simulink model "conv5x5_video_ex"  (Simulink 7.7)
settings: Solver=VariableStepDiscrete  SolverMode=SingleTasking  StartTime=0.0  StopTime=1000  RelTol=1e-3
undefined symbols (not defined in the file or in its folder): xrbsImage_r3
libraries: xbsIndex_r4 x204, xrbsImage_r4 x1, xbsCopyrightNotice_r4 x1
(part 1 of 3)
settings Model: Creator=alexc  LastModifiedBy=douangp
settings DataIOCC: SignalLoggingName=sigsOut
settings OptimizationCC: InlineParams=on  InitFltsAndDblsToZero=on
settings DebuggingCC: SaveWithParameterizedLinksMsg=none  SignalResolutionControl=TryResolveAllWithWarning  SolverPrmCheckMsg=none  MultiTaskDSMMsg=warning  MultiTaskCondExecSysMsg=none  StrictBusMsg=None
settings HardwareCC: TargetUnknown=on
settings RTWCC: IncludeERTFirstTime=on
settings GRTTargetCC: TargetFcnLib=ansi_tfl_tmw.mat

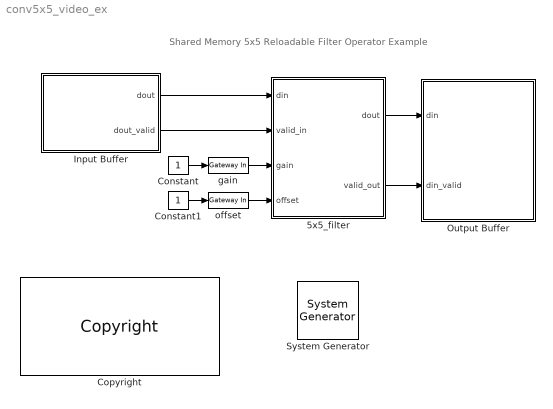
== system conv5x5_video_ex ==
  note: Shared Memory 5x5 Reloadable Filter Operator Example
  " System Generator" : xbsIndex_r4/ System Generator  Tag=genX  SystemSampleTime=-1  xilinxfamily=kintex7  part=xc7k325t  speed=-2  package=ffg900  synthesis_tool=XST  clock_wrapper=Clock Enables  directory=./netlist  proj_type=Project Navigator  Synth_file=XST Defaults  Impl_file=ISE Defaults  testbench=off  simulink_period=1/5  sysclk_period=20  dcm_input_clock_period=100  incr_netlist=off  trim_vbits=Everywhere in SubSystem  dbl_ovrd=According to Block Masks  core_generation=According to Block Masks  run_coregen=off  deprecated_control=off  eval_field=0  block_type=sysgen
      settings: block_version=9.2.00
  5x5_filter : Subsystem
  Constant : Constant
  Constant1 : Constant
  Copyright : xbsCopyrightNotice_r4/Copyright  copyrighttext="Copyright (c) 2011  by  Xilinx, Inc. All rights reserved.<br><br>This file contains proprietary, confidential information of Xilinx, Inc., is distributed under license from Xilinx, Inc., and may be used, copied and/or disclosed only pursuant to the terms of a valid license agreement with Xilinx, Inc. Xilinx hereby grants you a license to use this file solely for design, simulation, implementation and creation of design files limited to Xilinx devices or technologies. Use with non-Xilinx devices or technologies is expressly prohibited and immediately terminates your license unless covered by a separate agreement.<br><br>Xilinx is providing this design, code, or information \"as-is\" solely for use in developing programs and solutions for Xilinx devices, with no obligation on the part of Xilinx to provide support. By providing this design, code, or information as one possible implementation of this feature, application or standard, Xilinx is making no representation that this implementation is free from any claims of infringement. You are responsible for obtaining any rights you may require for your implementation. Xilinx expressly disclaims any warranty whatsoever with respect to the adequacy of the implementation, including but not limited to any warranties or representations that this implementation is free from claims of infringement, implied warranties of merchantability or fitness for a particular purpose.<br><br>Xilinx products are not intended for use in life support appliances, devices, or systems. Use in such applications is expressly prohibited.<br><br>Any modifications that are made to the Source Code are done at the user's sole risk and will be unsupported.<br><br>This copyright and support notice must be retained as part of this text at all times. (c) Copyright 1995-2011 Xilinx, Inc. All rights reserved."  block_type=copyright
      settings: block_version=10.1.00
      settings: infoedit=|
      | Copyright(C) 2008 by  Xilinx, Inc. All rights reserved.<br>
      | <br>
      | This file contains proprietary, confidential information of Xilinx, Inc., is distributed under license
      | from Xilinx, Inc., and may be used, copied and/or disclosed only pursuant to the terms of a valid license
      | agreement with Xilinx, Inc. Xilinx hereby grants you a license to use this file solely for design,
      | simulation, implementation and creation of design files limited to Xilinx devices or technologies. Use
      | with non-Xilinx devices or technologies is expressly prohibited and immediately terminates your license
      | unless covered by a separate agreement.<br>
      | <br>
      | Xilinx is providing this design, code, or information "as-is" solely for use in developing programs and
      | solutions for Xilinx devices, with no obligation on the part of Xilinx to provide support. By providing
      | this design, code, or information as one possible implementation of this feature, application or standard,
      | Xilinx is making no representation that this implementation is free from any claims of infringement. You
      | are responsible for obtaining any rights you may require for your implementation. Xilinx expressly disclaims
      | any warranty whatsoever with respect to the adequacy of the implementation, including but not limited to any
      | warranties or representations that this implementation is free from claims of infringement, implied warranties
      | of merchantability or fitness for a particular purpose.<br>
      | <br>
      | Xilinx products are not intended for use in life support appliances, devices, or systems. Use in such
      | applications is expressly prohibited.<br>
      | <br>
      | Any modifications that are made to the Source Code are done at the user's sole risk and will be unsupported.<br>
      | <br>
      | This copyright and support notice must be retained as part of this text at all times.
      | (c) Copyright 1995-2008 Xilinx, Inc. All rights reserved.
  Input Buffer : Subsystem  mask{smName='Foo', smDepth=128*128, smWidth=8}
      mask prompts: smName "Shared Memory Name"; smDepth "Shared Memory Depth"; smWidth "Shared Memory Width"
  Output Buffer : Subsystem  mask{smName='Bar', smDepth=128*128}
      mask prompts: smName "Shared Memory Name"; smDepth "Shared Memory Depth"
  gain : xbsIndex_r4/Gateway In  gui_display_data_type=Fixed-point  arith_type="Signed  (2's comp)"  n_bits=20  bin_pt=17  preci_type=Single  exp_width=8  frac_width=24  quantization="Round  (unbiased: +/- Inf)"  overflow=Saturate  period=1  dbl_ovrd=off  timing_constraint=None  locs_specified=off  LOCs={}  hdl_port=on  block_type=gatewayin
      settings: infoedit="Gateway in block.  Converts inputs of type Simulink integer, double and fixed point to  Xilinx fixed point type.<P><P>Hardware notes:  In hardware these blocks become top level input ports."  xl_area=[0, 0, 0, 0, 0, 0, 0]  block_version=VER_STRING_GOES_HERE
  offset : xbsIndex_r4/Gateway In  gui_display_data_type=Fixed-point  arith_type=Unsigned  n_bits=10  bin_pt=0  preci_type=Single  exp_width=8  frac_width=24  quantization="Round  (unbiased: +/- Inf)"  overflow=Saturate  period=1  dbl_ovrd=off  timing_constraint=None  locs_specified=off  LOCs={}  hdl_port=on  block_type=gatewayin
      settings: infoedit="Gateway in block.  Converts inputs of type Simulink integer, double and fixed point to  Xilinx fixed point type.<P><P>Hardware notes:  In hardware these blocks become top level input ports."  xl_area=[0, 0, 0, 0, 0, 0, 0]  block_version=VER_STRING_GOES_HERE
  wires:
  Input Buffer/1(dout) -> 5x5_filter/1(din)
  Constant/1 -> gain/1
  Constant1/1 -> offset/1
  5x5_filter/1(dout) -> Output Buffer/1(din)
  5x5_filter/2(valid_out) -> Output Buffer/2(din_valid)
  Input Buffer/2(dout_valid) -> 5x5_filter/2(valid_in)
  gain/1 -> 5x5_filter/3(gain)
  offset/1 -> 5x5_filter/4(offset)

== system conv5x5_video_ex/5x5_filter ==
  din : Inport
  valid_in : Inport  Port=2
  gain : Inport  Port=3
  offset : Inport  Port=4
  5x5Filter : Subsystem  AncestorBlock=xrbsImage_r3/5x5Filter  mask(5x5 Filter){maskNum=Smooth, coef_n_bits=6, coef_bin_pt=0, smpl_n_bits=8, smpl_bin_pt=0, smpl_period=1, maskVal=0, maskDiv=0}
      mask prompts: maskNum "5x5 Mask"; coef_n_bits "Number of Bits per Coefficient"; coef_bin_pt "Binary Point for Coefficient"; smpl_n_bits "Number of Bits per Input Sample"; smpl_bin_pt "Binary Point for Input Samples"; smpl_period "Sample Period"; maskVal "Mask Value"; maskDiv "Mask Division"
      mask help: The Xilinx 5x5 Filter reference block is implemented using 5 n-tap MAC FIR Filters. Nine different 2-D filters have been provided to filter grayscale images.
      mask init:
      | [bg,fg] = xlcmap('XBlock',0);
      | iPos = get_param(gcb,'Position');
      | iWidth=iPos(3)-iPos(1); iHeight=iPos(4)-iPos(2);
      | iCx=iWidth/2;
      | iCy=iHeight/2;
      | [logoX, logoY] = xlogo(iPos);
      | 
      | % Different 5x5 Filters 
      | %  by default edge is used
      | 
      | edge = [ 0  0  0  0 0; ...
      |          0 -1 -1 -1 0; ...
      |          0 -1  8 -1 0; ...
      |          0 -1 -1 -1 0; ...
      |          0  0  0  0 0];
      | edgeDiv = 1;
      | 
      | sobelX = [ 0  0  0  0 0; ...
      |            0 -1  0  1 0; ...
      |            0 -2  0  2 0; ...
      |            0 -1  0  1 0; ...
      |            0  0  0  0 0];
      | sobelXDiv = 1;
      | 
      | sobelY = [ 0  0  0  0 0; ...
      |            0  1  2  1 0; ...
      |            0  0  0  0 0; ...
      |            0 -1  2 -1 0; ...
      |            0  0  0  0 0];
      | sobelYDiv = 1;
      | 
      | sobelXY = [ 0  0  0  0 0; ...
      |             0  0 -1 -1 0; ...
      |             0  1  0 -1 0; ...
      |             0  1  1  0 0; ...
      |             0  0  0  0 0];
      | sobelXYDiv = 1;
      | 
      | blur = [ 1  1  1  1 1; ...
      |          1  0  0  0 1; ...
      |          1  0  0  0 1; ...
      |          1  0  0  0 1; ...
      |          1  1  1  1 1];
      | blurDiv = 1/16;
      | 
      | smooth = [ 1  1  1  1 1; ...
      |            1  5  5  5 1; ...
      |            1  5 44  5 1; ...
      |            1  5  5  5 1; ...
      |            1  1  1  1 1];
      | smoothDiv = 1/100;
      | 
      | sharpen = [ 0  0  0  0 0; ...
      |             0 -2 -2 -2 0; ...
      |             0 -2 32 -2 0; ...
      |             0 -2 -2 -2 0; ...
      |             0  0  0  0 0];
      | sharpenDiv = 1/16;
      | 
      | 
      | gaussian = [1 1 2 1 1; ...
      |             1 2 4 2 1; ...
      |             2 4 8 4 2; ...
      |             1 2 4 2 1; ...
      |             1 1 2 1 1];
      | gaussianDiv = 1/52;
      | 
      | identity = [ 0  0  0  0 0; ...
      |              0  0  0  0 0; ...
      |              0  0  1  0 0; ...
      |              0  0  0  0 0; ...
      |              0  0  0  0 0];
      | identityDiv = 1;
      | 
      | maskVal = zeros(5,5,5);
      | maskVal(:,:,1) = edge;
      | maskVal(:,:,2) = sobelX;
      | maskVal(:,:,3) = sobelY;
      | maskVal(:,:,4) = sobelXY;
      | maskVal(:,:,5) = blur;
      | maskVal(:,:,6) = smooth;
      | maskVal(:,:,7) = sharpen;
      | maskVal(:,:,8) = gaussian;
      | maskVal(:,:,9) = identity;
      | 
      | maskDiv = [edgeDiv sobelXDiv sobelYDiv sobelXYDiv blurDiv smoothDiv sharpenDiv gaussianDiv identityDiv];
      mask Help: web(xlhtmldoclink('5x5Filter'));
      mask StyleString: popup(Edge|Sobel X|Sobel Y|Sobel X-Y|Blur|Smooth|Sharpen|Gaussian|Identity),edit,edit,edit,edit,edit,edit,edit
      mask Display:
      | patch([0 iWidth iWidth 0],[0 0 iHeight iHeight] , bg);
      | patch(logoX,logoY , fg);
      | port_label('input',1,'Line1');
      | port_label('input',2,'Line2');
      | port_label('input',3,'Line3');
      | port_label('input',4,'Line4');
      | port_label('input',5,'Line5');
      | port_label('input',6,'Load');
      | port_label('input',7,'Coef');
      | port_label('input',8,'Gain');
      | port_label('output',1,'out');
      | plot([0 0 iWidth iWidth 0], [0 iHeight iHeight 0 0]);
  Register16 : xbsIndex_r4/Register  init=0  rst=off  en=off  dbl_ovrd=off  block_type=register
      settings: xl_area=[4 8 0 0 0 0 0]  block_version=VER_STRING_GOES_HERE
  Register2 : xbsIndex_r4/Register  init=0  rst=off  en=off  dbl_ovrd=off  block_type=register
      settings: xl_area=[4 8 0 0 0 0 0]  block_version=VER_STRING_GOES_HERE
  Virtex2 5 Line Buffer1 : xrbsImage_r4/Virtex2 5 Line Buffer  SystemSampleTime=-1  line_size=128  cst=1
      link override Virtex2 Line Buffer/Single Port RAM: block_version=8.2
      link override Virtex2 Line Buffer1/Single Port RAM: block_version=8.2
      link override Virtex2 Line Buffer2/Single Port RAM: block_version=8.2
      link override Virtex2 Line Buffer3/Single Port RAM: block_version=8.2
  coefficient_memory : Subsystem  mask{width=6, bin_pt=0, period=1/5}
      mask prompts: width "Coefficient Width"; bin_pt "Coefficient Binary Point"; period "Sample Period"
  valid_generator : Subsystem
  dout : Outport
  valid_out : Outport  Port=2
  wires:
  valid_in/1 -> valid_generator/1(valid_in)
  Register16/1 -> Virtex2 5 Line Buffer1/1
  5x5Filter/1(Out1) -> Register2/1
  Virtex2 5 Line Buffer1/1 -> 5x5Filter/1(Line1)
  Virtex2 5 Line Buffer1/2 -> 5x5Filter/2(Line2)
  Virtex2 5 Line Buffer1/3 -> 5x5Filter/3(Line3)
  Virtex2 5 Line Buffer1/4 -> 5x5Filter/4(Line4)
  Virtex2 5 Line Buffer1/5 -> 5x5Filter/5(Line5)
  Register2/1 -> dout/1
  din/1 -> Register16/1
  offset/1 -> valid_generator/2(offset)
  valid_generator/1(valid_out) -> valid_out/1
  gain/1 -> 5x5Filter/8(gain)
  coefficient_memory/1(load) -> 5x5Filter/6(load)
  coefficient_memory/2(coef) -> 5x5Filter/7(coef)

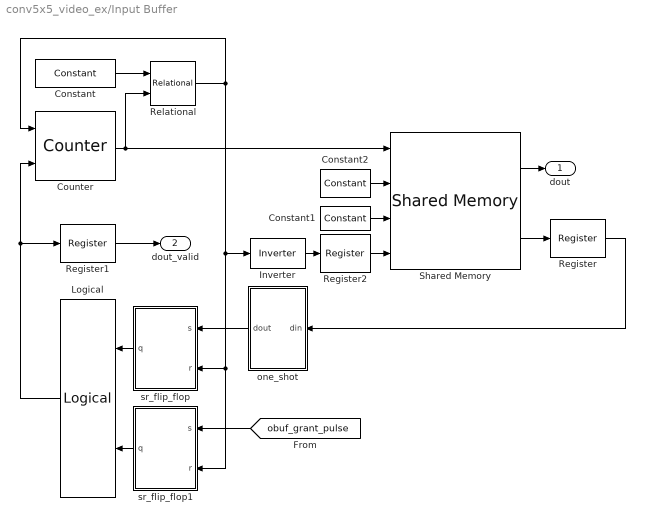
== system conv5x5_video_ex/Input Buffer ==
  Constant : xbsIndex_r4/Constant  const=smDepth-1  gui_display_data_type=Fixed-point  arith_type=Unsigned  n_bits=ceil(log2(smDepth))  bin_pt=0  preci_type=Single  exp_width=8  frac_width=24  explicit_period=on  period=1  equ=P=C  opselect=C  inp2=PCIN>>17  opr=+  inp1=P  carry=CIN  dbl_ovrd=off  block_type=constant
      settings: block_version=VER_STRING_GOES_HERE
  Constant1 : xbsIndex_r4/Constant  const=0  gui_display_data_type=Fixed-point  arith_type=Boolean  n_bits=1  bin_pt=0  preci_type=Single  exp_width=8  frac_width=24  explicit_period=off  period=1  equ=P=C  opselect=C  inp2=PCIN>>17  opr=+  inp1=P  carry=CIN  dbl_ovrd=off  block_type=constant
      settings: block_version=VER_STRING_GOES_HERE
  Constant2 : xbsIndex_r4/Constant  const=0  gui_display_data_type=Fixed-point  arith_type=Unsigned  n_bits=smWidth  bin_pt=0  preci_type=Single  exp_width=8  frac_width=24  explicit_period=off  period=1  equ=P=C  opselect=C  inp2=PCIN>>17  opr=+  inp1=P  carry=CIN  dbl_ovrd=off  block_type=constant
      settings: block_version=VER_STRING_GOES_HERE
  Counter : xbsIndex_r4/Counter  cnt_type=Free Running  cnt_to=Inf  operation=Up  start_count=0  cnt_by_val=1  arith_type=Unsigned  n_bits=ceil(log2(smDepth))  bin_pt=0  load_pin=off  rst=on  en=on  explicit_period=on  period=1  dbl_ovrd=off  use_behavioral_HDL=off  implementation=Fabric  use_rpm=off  block_type=counter
      settings: infoedit="Configurable up, down and up/down counter.<P><P>Hardware notes: Free running counters are the least expensive in hardware.  A count limited counter is implemented by combining a counter with a comparator."  xl_area=[0, 0, 0, 0, 0, 0, 0]  block_version=VER_STRING_GOES_HERE
  Inverter : xbsIndex_r4/Inverter  en=off  latency=0  dbl_ovrd=off  block_type=inv
      settings: xl_area=[0, 0, 0, 0, 0, 0, 0]  block_version=VER_STRING_GOES_HERE
  Logical : xbsIndex_r4/Logical  logical_function=AND  inputs=2  en=off  latency=0  precision=Full  arith_type=Unsigned  n_bits=8  bin_pt=2  align_bp=on  dbl_ovrd=off  block_type=logical
      settings: xl_area=[0, 0, 0, 0, 0, 0, 0]  block_version=VER_STRING_GOES_HERE
  Register : xbsIndex_r4/Register  init=0  rst=off  en=off  dbl_ovrd=off  block_type=register
      settings: xl_area=[0, 0, 0, 0, 0, 0, 0]  block_version=VER_STRING_GOES_HERE
  Register1 : xbsIndex_r4/Register  init=0  rst=off  en=off  dbl_ovrd=off  block_type=register
      settings: xl_area=[0, 0, 0, 0, 0, 0, 0]  block_version=VER_STRING_GOES_HERE
  Register2 : xbsIndex_r4/Register  init=0  rst=off  en=off  dbl_ovrd=off  block_type=register
      settings: xl_area=[0, 0, 0, 0, 0, 0, 0]  block_version=VER_STRING_GOES_HERE
  Relational : xbsIndex_r4/Relational  mode=a=b  en=off  latency=0  dbl_ovrd=off  block_type=relational
      settings: xl_area=[0, 0, 0, 0, 0, 0, 0]  block_version=VER_STRING_GOES_HERE
  Shared Memory : xbsIndex_r4/Shared Memory  shared_memory_name=smName  depth=smDepth  ownership=Locally Owned and Initialized  initVector=0:255  en=off  mutex=Lockable  mode=Read and Write  write_mode=Read After Write  time_out=0  latency=1  explicit_data_type=off  gui_display_data_type=Fixed-point  arith_type=Unsigned  n_bits=0  bin_pt=0  preci_type=Single  implementation=Block RAM  use_rpm=off  block_type=shmem
      settings: AttributesFormatString=<< %<shared_memory_name> >>  xl_area=[0, 0, 0, 0, 0, 0, 0]  block_version=VER_STRING_GOES_HERE
  one_shot : Subsystem
  sr_flip_flop : Subsystem
  sr_flip_flop1 : Subsystem
  dout : Outport
  dout_valid : Outport  Port=2
  wires:
  Shared Memory/2 -> Register/1
  Counter/1 -> Shared Memory/1, Relational/2
  Constant/1 -> Relational/1
  Relational/1 -> Inverter/1, sr_flip_flop/2(r), sr_flip_flop1/2(r), Counter/1
  Inverter/1 -> Register2/1
  Register2/1 -> Shared Memory/4
  Constant1/1 -> Shared Memory/3
  Constant2/1 -> Shared Memory/2
  [obuf_grant_pulse] -> sr_flip_flop1/1(s)
  one_shot/1(dout) -> sr_flip_flop/1(s)
  sr_flip_flop1/1(q) -> Logical/2
  sr_flip_flop/1(q) -> Logical/1
  Logical/1 -> Counter/2, Register1/1
  Register/1 -> one_shot/1(din)
  Register1/1 -> dout_valid/1
  Shared Memory/1 -> dout/1

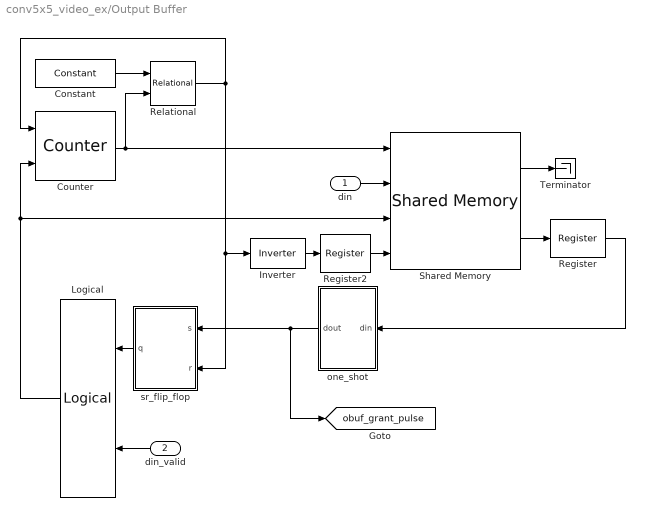
== system conv5x5_video_ex/Output Buffer ==
  din : Inport
  din_valid : Inport  Port=2
  Constant : xbsIndex_r4/Constant  const=smDepth-1  gui_display_data_type=Fixed-point  arith_type=Unsigned  n_bits=ceil(log2(smDepth))  bin_pt=0  preci_type=Single  exp_width=8  frac_width=24  explicit_period=on  period=1  equ=P=C  opselect=C  inp2=PCIN>>17  opr=+  inp1=P  carry=CIN  dbl_ovrd=off  block_type=constant
      settings: block_version=VER_STRING_GOES_HERE
  Counter : xbsIndex_r4/Counter  cnt_type=Free Running  cnt_to=Inf  operation=Up  start_count=0  cnt_by_val=1  arith_type=Unsigned  n_bits=ceil(log2(smDepth))  bin_pt=0  load_pin=off  rst=on  en=on  explicit_period=on  period=1  dbl_ovrd=off  use_behavioral_HDL=off  implementation=Fabric  use_rpm=off  block_type=counter
      settings: infoedit="Configurable up, down and up/down counter.<P><P>Hardware notes: Free running counters are the least expensive in hardware.  A count limited counter is implemented by combining a counter with a comparator."  xl_area=[0, 0, 0, 0, 0, 0, 0]  block_version=VER_STRING_GOES_HERE
  Inverter : xbsIndex_r4/Inverter  en=off  latency=0  dbl_ovrd=off  block_type=inv
      settings: xl_area=[0, 0, 0, 0, 0, 0, 0]  block_version=VER_STRING_GOES_HERE
  Logical : xbsIndex_r4/Logical  logical_function=AND  inputs=2  en=off  latency=0  precision=Full  arith_type=Unsigned  n_bits=8  bin_pt=2  align_bp=on  dbl_ovrd=off  block_type=logical
      settings: xl_area=[0, 0, 0, 0, 0, 0, 0]  block_version=VER_STRING_GOES_HERE
  Register : xbsIndex_r4/Register  init=0  rst=off  en=off  dbl_ovrd=off  block_type=register
      settings: xl_area=[0, 0, 0, 0, 0, 0, 0]  block_version=VER_STRING_GOES_HERE
  Register2 : xbsIndex_r4/Register  init=0  rst=off  en=off  dbl_ovrd=off  block_type=register
      settings: xl_area=[0, 0, 0, 0, 0, 0, 0]  block_version=VER_STRING_GOES_HERE
  Relational : xbsIndex_r4/Relational  mode=a=b  en=off  latency=0  dbl_ovrd=off  block_type=relational
      settings: xl_area=[0, 0, 0, 0, 0, 0, 0]  block_version=VER_STRING_GOES_HERE
  Shared Memory : xbsIndex_r4/Shared Memory  shared_memory_name=smName  depth=smDepth  ownership=Locally Owned and Initialized  initVector=0  en=off  mutex=Lockable  mode=Read and Write  write_mode=Read After Write  time_out=0  latency=1  explicit_data_type=off  gui_display_data_type=Fixed-point  arith_type=Unsigned  n_bits=0  bin_pt=0  preci_type=Single  implementation=Block RAM  use_rpm=off  block_type=shmem
      settings: AttributesFormatString=<< %<shared_memory_name> >>  xl_area=[0, 0, 0, 0, 0, 0, 0]  block_version=VER_STRING_GOES_HERE
  Terminator : Terminator
  one_shot : Subsystem
  sr_flip_flop : Subsystem
  tag scope: obuf_grant_pulse=global
  wires:
  Shared Memory/1 -> Terminator/1
  Register/1 -> one_shot/1(din)
  Logical/1 -> Counter/2, Shared Memory/3
  sr_flip_flop/1(q) -> Logical/1
  one_shot/1(dout) -> sr_flip_flop/1(s), [obuf_grant_pulse]
  Register2/1 -> Shared Memory/4
  Inverter/1 -> Register2/1
  Relational/1 -> Counter/1, Inverter/1, sr_flip_flop/2(r)
  Constant/1 -> Relational/1
  Counter/1 -> Relational/2, Shared Memory/1
  Shared Memory/2 -> Register/1
  din_valid/1 -> Logical/2
  din/1 -> Shared Memory/2

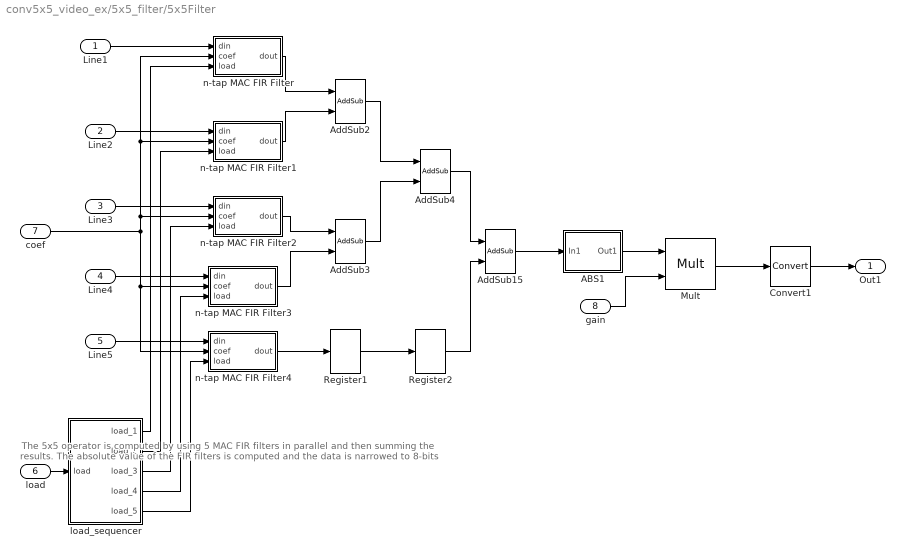
== system conv5x5_video_ex/5x5_filter/5x5Filter ==
  note: The 5x5 operator is computed by using 5 MAC FIR filters in parallel and then
      | summing the results.  The absolute value of the FIR filters is computed
      | and the data is narrowed to 8-bits
  Line1 : Inport
  Line2 : Inport  Port=2
  Line3 : Inport  Port=3
  Line4 : Inport  Port=4
  Line5 : Inport  Port=5
  load : Inport  Port=6
  coef : Inport  Port=7
  gain : Inport  Port=8
  ABS1 : Subsystem
  AddSub{2..4,15} (4 alike) : xbsIndex_r4/AddSub  mode=Addition  use_carryin=off  use_carryout=off  en=off  latency=1  precision=Full  arith_type=Unsigned  n_bits=8  bin_pt=2  quantization=Truncate  overflow=Wrap  dbl_ovrd=off  use_behavioral_HDL=off  hw_selection=Fabric  pipelined=off  use_rpm=off  block_type=addsub
      settings: xl_area=[0, 0, 0, 0, 0, 0, 0]  block_version=VER_STRING_GOES_HERE
  Convert1 : xbsIndex_r4/Convert  gui_display_data_type=Fixed-point  arith_type=Unsigned  n_bits=8  bin_pt=0  float_type=Single  exp_bits=8  fraction_bits=24  quantization=Truncate  overflow=Saturate  en=off  latency=1  dbl_ovrd=off  pipeline=off  block_type=convert
      settings: infoedit=The input is presented at the output after quantization and overflow effects.<P><P>Hardware notes: Additional hardware is used when rounding or saturation is selected and output width is less than the input width.  xl_area=[0, 0, 0, 0, 0, 0, 0]  block_version=VER_STRING_GOES_HERE
  Mult : xbsIndex_r4/Mult  precision=Full  arith_type="Signed  (2's comp)"  n_bits=8  bin_pt=2  quantization=Truncate  overflow=Wrap  en=off  latency=5  dbl_ovrd=off  use_behavioral_HDL=off  opt=Speed  use_embedded=on  optimum_pipeline=off  pipeline=on  use_rpm=off  placement_style=Rectangular shape  block_type=mult
      settings: infoedit=Multiplies two values.<P><P>Hardware notes: To use the internal pipeline stage of the dedicated multiplier you must select 'Pipeline to Greatest Extent Possible'.  xl_area=[0, 0, 0, 0, 0, 0, 0]  block_version=VER_STRING_GOES_HERE
  Register1 : xbsIndex_r4/Register  init=0  rst=off  en=off  dbl_ovrd=off  block_type=register
      settings: xl_area=[0, 0, 0, 0, 0, 0, 0]  block_version=VER_STRING_GOES_HERE
  Register2 : xbsIndex_r4/Register  init=0  rst=off  en=off  dbl_ovrd=off  block_type=register
      settings: xl_area=[0, 0, 0, 0, 0, 0, 0]  block_version=VER_STRING_GOES_HERE
  load_sequencer : Subsystem  mask{num_coef=5}
      mask prompts: num_coef "Number of Coefficients"
  n-tap MAC FIR Filter : Subsystem  AncestorBlock=xrbsDSP_r3/n-tap MAC FIR Filter  mask(n-tap MAC FIR Filter){coef=maskVal(1,5:-1:1,maskNum), coef_n_bits=coef_n_bits, coef_bin_pt=coef_bin_pt, smpl_n_bits=smpl_n_bits, smpl_bin_pt=smpl_bin_pt, smpl_period=smpl_period}
      mask prompts: coef "Coefficients"; coef_n_bits "Number of Bits per Coefficient"; coef_bin_pt "Binary Point for Coefficient"; smpl_n_bits "Number of Bits per Input Sample"; smpl_bin_pt "Binary Point for Input Samples"; smpl_period "Input Sample Period"
      mask help: MAC-based FIR filter with n coefficients.
      mask init:
      | dstr = sprintf('%d tap',length(coef));
      | 
      | [bg,fg] = xlcmap('XBlock',0);
      | iPos = get_param(gcb,'Position');
      | iWidth=iPos(3)-iPos(1); iHeight=iPos(4)-iPos(2);
      | iCx=iWidth/2;
      | iCy=iHeight/2;
      | [logoX, logoY] = xlogo(iPos);
      mask Help: web(xlhtmldoclink('n-tap MAC FIR Filter'));
      mask Display:
      | patch([0 iWidth iWidth 0],[0 0 iHeight iHeight] , bg);
      | patch(logoX,logoY, fg);
      | text(iCx/1.8,iCy+2,dstr);
      | text(iCx/2.0-4,iCy-10,'MAC FIR');
      | plot([0 0 iWidth iWidth 0], [0 iHeight iHeight 0 0]);
  n-tap MAC FIR Filter1 : Subsystem  AncestorBlock=xrbsDSP_r3/n-tap MAC FIR Filter  mask(n-tap MAC FIR Filter){coef=maskVal(2,5:-1:1,maskNum), coef_n_bits=coef_n_bits, coef_bin_pt=coef_bin_pt, smpl_n_bits=smpl_n_bits, smpl_bin_pt=smpl_bin_pt, smpl_period=smpl_period}
      mask prompts: coef "Coefficients"; coef_n_bits "Number of Bits per Coefficient"; coef_bin_pt "Binary Point for Coefficient"; smpl_n_bits "Number of Bits per Input Sample"; smpl_bin_pt "Binary Point for Input Samples"; smpl_period "Input Sample Period"
      mask help: MAC-based FIR filter with n coefficients.
      mask init: same as conv5x5_video_ex/5x5_filter/5x5Filter/n-tap MAC FIR Filter
      mask Help: web(xlhtmldoclink('n-tap MAC FIR Filter'));
      mask Display:
      | patch([0 iWidth iWidth 0],[0 0 iHeight iHeight] , bg);
      | patch(logoX,logoY, fg);
      | text(iCx/1.8,iCy+2,dstr);
      | text(iCx/2.0-4,iCy-10,'MAC FIR');
      | plot([0 0 iWidth iWidth 0], [0 iHeight iHeight 0 0]);
  n-tap MAC FIR Filter2 : Subsystem  AncestorBlock=xrbsDSP_r3/n-tap MAC FIR Filter  mask(n-tap MAC FIR Filter){coef=maskVal(3,5:-1:1,maskNum), coef_n_bits=coef_n_bits, coef_bin_pt=coef_bin_pt, smpl_n_bits=smpl_n_bits, smpl_bin_pt=smpl_bin_pt, smpl_period=smpl_period}
      mask prompts: coef "Coefficients"; coef_n_bits "Number of Bits per Coefficient"; coef_bin_pt "Binary Point for Coefficient"; smpl_n_bits "Number of Bits per Input Sample"; smpl_bin_pt "Binary Point for Input Samples"; smpl_period "Input Sample Period"
      mask help: MAC-based FIR filter with n coefficients.
      mask init: same as conv5x5_video_ex/5x5_filter/5x5Filter/n-tap MAC FIR Filter
      mask Help: web(xlhtmldoclink('n-tap MAC FIR Filter'));
      mask Display:
      | patch([0 iWidth iWidth 0],[0 0 iHeight iHeight] , bg);
      | patch(logoX,logoY, fg);
      | text(iCx/1.8,iCy+2,dstr);
      | text(iCx/2.0-4,iCy-10,'MAC FIR');
      | plot([0 0 iWidth iWidth 0], [0 iHeight iHeight 0 0]);
  n-tap MAC FIR Filter3 : Subsystem  AncestorBlock=xrbsDSP_r3/n-tap MAC FIR Filter  mask(n-tap MAC FIR Filter){coef=maskVal(4,5:-1:1,maskNum), coef_n_bits=coef_n_bits, coef_bin_pt=coef_bin_pt, smpl_n_bits=smpl_n_bits, smpl_bin_pt=smpl_bin_pt, smpl_period=smpl_period}
      mask prompts: coef "Coefficients"; coef_n_bits "Number of Bits per Coefficient"; coef_bin_pt "Binary Point for Coefficient"; smpl_n_bits "Number of Bits per Input Sample"; smpl_bin_pt "Binary Point for Input Samples"; smpl_period "Input Sample Period"
      mask help: MAC-based FIR filter with n coefficients.
      mask init: same as conv5x5_video_ex/5x5_filter/5x5Filter/n-tap MAC FIR Filter
      mask Help: web(xlhtmldoclink('n-tap MAC FIR Filter'));
      mask Display:
      | patch([0 iWidth iWidth 0],[0 0 iHeight iHeight] , bg);
      | patch(logoX,logoY, fg);
      | text(iCx/1.8,iCy+2,dstr);
      | text(iCx/2.0-4,iCy-10,'MAC FIR');
      | plot([0 0 iWidth iWidth 0], [0 iHeight iHeight 0 0]);
  n-tap MAC FIR Filter4 : Subsystem  AncestorBlock=xrbsDSP_r3/n-tap MAC FIR Filter  mask(n-tap MAC FIR Filter){coef=maskVal(5,5:-1:1,maskNum), coef_n_bits=coef_n_bits, coef_bin_pt=coef_bin_pt, smpl_n_bits=smpl_n_bits, smpl_bin_pt=smpl_bin_pt, smpl_period=smpl_period}
      mask prompts: coef "Coefficients"; coef_n_bits "Number of Bits per Coefficient"; coef_bin_pt "Binary Point for Coefficient"; smpl_n_bits "Number of Bits per Input Sample"; smpl_bin_pt "Binary Point for Input Samples"; smpl_period "Input Sample Period"
      mask help: MAC-based FIR filter with n coefficients.
      mask init: same as conv5x5_video_ex/5x5_filter/5x5Filter/n-tap MAC FIR Filter
      mask Help: web(xlhtmldoclink('n-tap MAC FIR Filter'));
      mask Display:
      | patch([0 iWidth iWidth 0],[0 0 iHeight iHeight] , bg);
      | patch(logoX,logoY, fg);
      | text(iCx/1.8,iCy+2,dstr);
      | text(iCx/2.0-4,iCy-10,'MAC FIR');
      | plot([0 0 iWidth iWidth 0], [0 iHeight iHeight 0 0]);
  Out1 : Outport
  wires:
  Line1/1 -> n-tap MAC FIR Filter/1(din)
  Line2/1 -> n-tap MAC FIR Filter1/1(din)
  Line4/1 -> n-tap MAC FIR Filter3/1(din)
  Line5/1 -> n-tap MAC FIR Filter4/1(din)
  n-tap MAC FIR Filter/1(dout) -> AddSub2/1
  n-tap MAC FIR Filter1/1(dout) -> AddSub2/2
  n-tap MAC FIR Filter2/1(dout) -> AddSub3/1
  n-tap MAC FIR Filter3/1(dout) -> AddSub3/2
  AddSub2/1 -> AddSub4/1
  AddSub3/1 -> AddSub4/2
  n-tap MAC FIR Filter4/1(dout) -> Register1/1
  Register1/1 -> Register2/1
  AddSub15/1 -> ABS1/1(In1)
  AddSub4/1 -> AddSub15/1
  Register2/1 -> AddSub15/2
  Mult/1 -> Convert1/1
  ABS1/1(Out1) -> Mult/1
  Convert1/1 -> Out1/1
  gain/1 -> Mult/2
  load/1 -> load_sequencer/1(load)
  Line3/1 -> n-tap MAC FIR Filter2/1(din)
  load_sequencer/1(load_1) -> n-tap MAC FIR Filter/3(load)
  load_sequencer/2(load_2) -> n-tap MAC FIR Filter1/3(load)
  load_sequencer/3(load_3) -> n-tap MAC FIR Filter2/3(load)
  load_sequencer/4(load_4) -> n-tap MAC FIR Filter3/3(load)
  load_sequencer/5(load_5) -> n-tap MAC FIR Filter4/3(load)
  coef/1 -> n-tap MAC FIR Filter/2(coef), n-tap MAC FIR Filter1/2(coef), n-tap MAC FIR Filter2/2(coef), n-tap MAC FIR Filter3/2(coef), n-tap MAC FIR Filter4/2(coef)

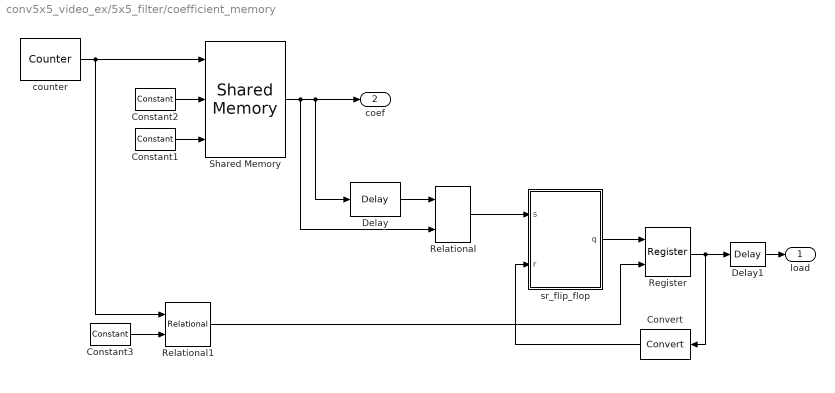
== system conv5x5_video_ex/5x5_filter/coefficient_memory ==
  Constant1 : xbsIndex_r4/Constant  const=0  gui_display_data_type=Fixed-point  arith_type=Boolean  n_bits=width  bin_pt=bin_pt  preci_type=Single  exp_width=8  frac_width=24  explicit_period=off  period=1  equ=P=C  opselect=C  inp2=PCIN>>17  opr=+  inp1=P  carry=CIN  dbl_ovrd=off  block_type=constant
      settings: block_version=VER_STRING_GOES_HERE
  Constant2 : xbsIndex_r4/Constant  const=0  gui_display_data_type=Fixed-point  arith_type=Signed (2's comp)  n_bits=width  bin_pt=bin_pt  preci_type=Single  exp_width=8  frac_width=24  explicit_period=off  period=1  equ=P=C  opselect=C  inp2=PCIN>>17  opr=+  inp1=P  carry=CIN  dbl_ovrd=off  block_type=constant
      settings: block_version=VER_STRING_GOES_HERE
  Constant3 : xbsIndex_r4/Constant  const=24  gui_display_data_type=Fixed-point  arith_type=Unsigned  n_bits=5  bin_pt=0  preci_type=Single  exp_width=8  frac_width=24  explicit_period=off  period=1  equ=P=C  opselect=C  inp2=PCIN>>17  opr=+  inp1=P  carry=CIN  dbl_ovrd=off  block_type=constant
      settings: block_version=VER_STRING_GOES_HERE
  Convert : xbsIndex_r4/Convert  gui_display_data_type=Fixed-point  arith_type=Boolean  n_bits=8  bin_pt=6  float_type=Single  exp_bits=8  fraction_bits=24  quantization=Truncate  overflow=Wrap  en=off  latency=0  dbl_ovrd=off  pipeline=off  block_type=convert
      settings: infoedit=The input is presented at the output after quantization and overflow effects.<P><P>Hardware notes: Additional hardware is used when rounding or saturation is selected and output width is less than the input width.  xl_area=[0, 0, 0, 0, 0, 0, 0]  block_version=VER_STRING_GOES_HERE
  Delay : xbsIndex_r4/Delay  rst=off  infoeditControl=Selection of Reset will increase slice count due to use of real FFs and instead of SRLs  en=off  latency=25  dbl_ovrd=off  reg_retiming=off  block_type=delay
      settings: infoedit="Delay line having  configurable length.<P><P>Hardware notes: A delay line is a chain, each link of which is an SRL16 followed by a flip-flop. If register retiming is enabled, the delay line is a chain of flip-flops."  xl_area=[0, 0, 0, 0, 0, 0, 0]  block_version=VER_STRING_GOES_HERE
  Delay1 : xbsIndex_r4/Delay  rst=off  infoeditControl=Selection of Reset will increase slice count due to use of real FFs and instead of SRLs  en=off  latency=1  dbl_ovrd=off  reg_retiming=off  block_type=delay
      settings: infoedit="Delay line having  configurable length.<P><P>Hardware notes: A delay line is a chain, each link of which is an SRL16 followed by a flip-flop. If register retiming is enabled, the delay line is a chain of flip-flops."  xl_area=[0, 0, 0, 0, 0, 0, 0]  block_version=VER_STRING_GOES_HERE
  Register : xbsIndex_r4/Register  init=0  rst=off  en=on  dbl_ovrd=off  block_type=register
      settings: xl_area=[0, 0, 0, 0, 0, 0, 0]  block_version=VER_STRING_GOES_HERE
  Relational : xbsIndex_r4/Relational  mode=a!=b  en=off  latency=0  dbl_ovrd=off  block_type=relational
      settings: xl_area=[0, 0, 0, 0, 0, 0, 0]  block_version=VER_STRING_GOES_HERE
  Relational1 : xbsIndex_r4/Relational  mode=a=b  en=off  latency=0  dbl_ovrd=off  block_type=relational
      settings: xl_area=[0, 0, 0, 0, 0, 0, 0]  block_version=VER_STRING_GOES_HERE
  Shared Memory : xbsIndex_r4/Shared Memory  shared_memory_name='coef_buffer'  depth=32  ownership=Locally Owned and Initialized  initVector=0  en=off  mutex=Unprotected  mode=Read and Write  write_mode=Read After Write  time_out=0  latency=1  explicit_data_type=off  gui_display_data_type=Fixed-point  arith_type=Unsigned  n_bits=0  bin_pt=0  preci_type=Single  implementation=Block RAM  use_rpm=off  block_type=shmem
      settings: AttributesFormatString=Shared as %<shared_memory_name>  xl_area=[0, 0, 0, 0, 0, 0, 0]  block_version=VER_STRING_GOES_HERE
  counter : xbsIndex_r4/Counter  cnt_type=Count Limited  cnt_to=24  operation=Up  start_count=0  cnt_by_val=1  arith_type=Unsigned  n_bits=5  bin_pt=0  load_pin=off  rst=off  en=off  explicit_period=on  period=period  dbl_ovrd=off  use_behavioral_HDL=off  implementation=Fabric  use_rpm=off  block_type=counter
      settings: infoedit="Configurable up, down and up/down counter.<P><P>Hardware notes: Free running counters are the least expensive in hardware.  A count limited counter is implemented by combining a counter with a comparator."  xl_area=[0, 0, 0, 0, 0, 0, 0]  block_version=VER_STRING_GOES_HERE
  sr_flip_flop : Subsystem
  load : Outport
  coef : Outport  Port=2
  wires:
  Register/1 -> Delay1/1, Convert/1
  Delay1/1 -> load/1
  sr_flip_flop/1(q) -> Register/1
  Relational1/1 -> Register/2
  Constant3/1 -> Relational1/2
  Relational/1 -> sr_flip_flop/1(s)
  Delay/1 -> Relational/1
  Shared Memory/1 -> Relational/2, coef/1, Delay/1
  Constant1/1 -> Shared Memory/3
  counter/1 -> Relational1/1, Shared Memory/1
  Constant2/1 -> Shared Memory/2
  Convert/1 -> sr_flip_flop/2(r)

== system conv5x5_video_ex/5x5_filter/valid_generator ==
  valid_in : Inport
  offset : Inport  Port=2
  ASR : xbsIndex_r4/Addressable Shift Register  infer_latency=on  depth=2  initVector=[0]  en=off  dbl_ovrd=off  use_behavioral_HDL=off  Optimization=Resource  use_rpm=on  block_type=addrsr
      settings: infoedit="Delay of configurable length.  Any element in the delay line can be addressed and driven onto the output port.<P><P>Hardware notes: Implemented using SRL16s.  If a Virtex-II device is used, multiple SRLC16s are cascaded together."  xl_area=[0, 0, 0, 0, 0, 0, 0]  block_version=VER_STRING_GOES_HERE
  Register : xbsIndex_r4/Register  init=0  rst=off  en=off  dbl_ovrd=off  block_type=register
      settings: xl_area=[0, 0, 0, 0, 0, 0, 0]  block_version=VER_STRING_GOES_HERE
  Register1 : xbsIndex_r4/Register  init=0  rst=off  en=on  dbl_ovrd=off  block_type=register
      settings: xl_area=[0, 0, 0, 0, 0, 0, 0]  block_version=VER_STRING_GOES_HERE
  one_shot : Subsystem
  valid_out : Outport
  wires:
  valid_in/1 -> Register/1, one_shot/1(din)
  Register/1 -> ASR/1
  ASR/1 -> valid_out/1
  Register1/1 -> ASR/2
  offset/1 -> Register1/1
  one_shot/1(dout) -> Register1/2

== system conv5x5_video_ex/Input Buffer/one_shot ==
  din : Inport
  Inverter : xbsIndex_r4/Inverter  en=off  latency=0  dbl_ovrd=off  block_type=inv
      settings: xl_area=[0, 0, 0, 0, 0, 0, 0]  block_version=VER_STRING_GOES_HERE
  Logical : xbsIndex_r4/Logical  logical_function=AND  inputs=2  en=off  latency=0  precision=Full  arith_type=Unsigned  n_bits=8  bin_pt=2  align_bp=on  dbl_ovrd=off  block_type=logical
      settings: xl_area=[0, 0, 0, 0, 0, 0, 0]  block_version=VER_STRING_GOES_HERE
  Register1 : xbsIndex_r4/Register  init=0  rst=off  en=off  dbl_ovrd=off  block_type=register
      settings: xl_area=[0, 0, 0, 0, 0, 0, 0]  block_version=VER_STRING_GOES_HERE
  dout : Outport
  wires:
  din/1 -> Register1/1, Logical/1
  Register1/1 -> Inverter/1
  Inverter/1 -> Logical/2
  Logical/1 -> dout/1

== system conv5x5_video_ex/Input Buffer/sr_flip_flop ==
  s : Inport
  r : Inport  Port=2
  Constant2 : xbsIndex_r4/Constant  const=1  gui_display_data_type=Fixed-point  arith_type=Boolean  n_bits=1  bin_pt=0  preci_type=Single  exp_width=8  frac_width=24  explicit_period=off  period=1  equ=P=C  opselect=C  inp2=PCIN>>17  opr=+  inp1=P  carry=CIN  dbl_ovrd=off  block_type=constant
      settings: block_version=VER_STRING_GOES_HERE
  Register1 : xbsIndex_r4/Register  init=0  rst=on  en=on  dbl_ovrd=off  block_type=register
      settings: xl_area=[0, 0, 0, 0, 0, 0, 0]  block_version=VER_STRING_GOES_HERE
  q : Outport
  wires:
  Register1/1 -> q/1
  Constant2/1 -> Register1/1
  r/1 -> Register1/2
  s/1 -> Register1/3

== system conv5x5_video_ex/Input Buffer/sr_flip_flop1 ==
  s : Inport
  r : Inport  Port=2
  Constant2 : xbsIndex_r4/Constant  const=1  gui_display_data_type=Fixed-point  arith_type=Boolean  n_bits=1  bin_pt=0  preci_type=Single  exp_width=8  frac_width=24  explicit_period=off  period=1  equ=P=C  opselect=C  inp2=PCIN>>17  opr=+  inp1=P  carry=CIN  dbl_ovrd=off  block_type=constant
      settings: block_version=VER_STRING_GOES_HERE
  Register1 : xbsIndex_r4/Register  init=0  rst=on  en=on  dbl_ovrd=off  block_type=register
      settings: xl_area=[0, 0, 0, 0, 0, 0, 0]  block_version=VER_STRING_GOES_HERE
  q : Outport
  wires:
  s/1 -> Register1/3
  r/1 -> Register1/2
  Constant2/1 -> Register1/1
  Register1/1 -> q/1

== system conv5x5_video_ex/Output Buffer/one_shot ==
  din : Inport
  Inverter : xbsIndex_r4/Inverter  en=off  latency=0  dbl_ovrd=off  block_type=inv
      settings: xl_area=[0, 0, 0, 0, 0, 0, 0]  block_version=VER_STRING_GOES_HERE
  Logical : xbsIndex_r4/Logical  logical_function=AND  inputs=2  en=off  latency=0  precision=Full  arith_type=Unsigned  n_bits=8  bin_pt=2  align_bp=on  dbl_ovrd=off  block_type=logical
      settings: xl_area=[0, 0, 0, 0, 0, 0, 0]  block_version=VER_STRING_GOES_HERE
  Register1 : xbsIndex_r4/Register  init=0  rst=off  en=off  dbl_ovrd=off  block_type=register
      settings: xl_area=[0, 0, 0, 0, 0, 0, 0]  block_version=VER_STRING_GOES_HERE
  dout : Outport
  wires:
  Logical/1 -> dout/1
  Inverter/1 -> Logical/2
  Register1/1 -> Inverter/1
  din/1 -> Logical/1, Register1/1

== system conv5x5_video_ex/Output Buffer/sr_flip_flop ==
  s : Inport
  r : Inport  Port=2
  Constant2 : xbsIndex_r4/Constant  const=1  gui_display_data_type=Fixed-point  arith_type=Boolean  n_bits=1  bin_pt=0  preci_type=Single  exp_width=8  frac_width=24  explicit_period=off  period=1  equ=P=C  opselect=C  inp2=PCIN>>17  opr=+  inp1=P  carry=CIN  dbl_ovrd=off  block_type=constant
      settings: block_version=VER_STRING_GOES_HERE
  Register1 : xbsIndex_r4/Register  init=0  rst=on  en=on  dbl_ovrd=off  block_type=register
      settings: xl_area=[0, 0, 0, 0, 0, 0, 0]  block_version=VER_STRING_GOES_HERE
  q : Outport
  wires:
  s/1 -> Register1/3
  r/1 -> Register1/2
  Constant2/1 -> Register1/1
  Register1/1 -> q/1

== system conv5x5_video_ex/5x5_filter/5x5Filter/ABS1 ==
  In1 : Inport
  Mux : xbsIndex_r4/Mux  inputs=2  en=off  latency=1  precision=Full  arith_type=Unsigned  n_bits=8  bin_pt=0  quantization=Truncate  overflow=Saturate  dbl_ovrd=off  block_type=mux
      settings: xl_area=[0, 0, 0, 0, 0, 0, 0]  block_version=VER_STRING_GOES_HERE
  Negate : xbsIndex_r4/Negate  precision=Full  arith_type=Unsigned  n_bits=8  bin_pt=2  quantization=Truncate  overflow=Wrap  en=off  latency=1  dbl_ovrd=off  block_type=negate
      settings: xl_area=[0, 0, 0, 0, 0, 0, 0]  block_version=VER_STRING_GOES_HERE
  Register1 : xbsIndex_r4/Register  init=0  rst=off  en=off  dbl_ovrd=off  block_type=register
      settings: xl_area=[0, 0, 0, 0, 0, 0, 0]  block_version=VER_STRING_GOES_HERE
  Register2 : xbsIndex_r4/Register  init=0  rst=off  en=off  dbl_ovrd=off  block_type=register
      settings: xl_area=[0, 0, 0, 0, 0, 0, 0]  block_version=VER_STRING_GOES_HERE
  Slice : xbsIndex_r4/Slice  nbits=1  boolean_output=off  mode=Upper Bit Location + Width  bit1=0  base1=MSB of Input  bit0=0  base0=LSB of Input  dbl_ovrd=off  block_type=slice
      settings: infoedit="Extracts a given range of bits from each input sample and presents it at the output.  The output type is ordinarily unsigned with binary point at zero, but can be Boolean when the slice is one bit wide.<P><P>Hardware notes: In hardware this block costs nothing."  block_version=VER_STRING_GOES_HERE
  Out1 : Outport
  wires:
  Register1/1 -> Mux/2
  Register2/1 -> Mux/1
  Mux/1 -> Out1/1
  In1/1 -> Register1/1, Slice/1, Negate/1
  Negate/1 -> Mux/3
  Slice/1 -> Register2/1

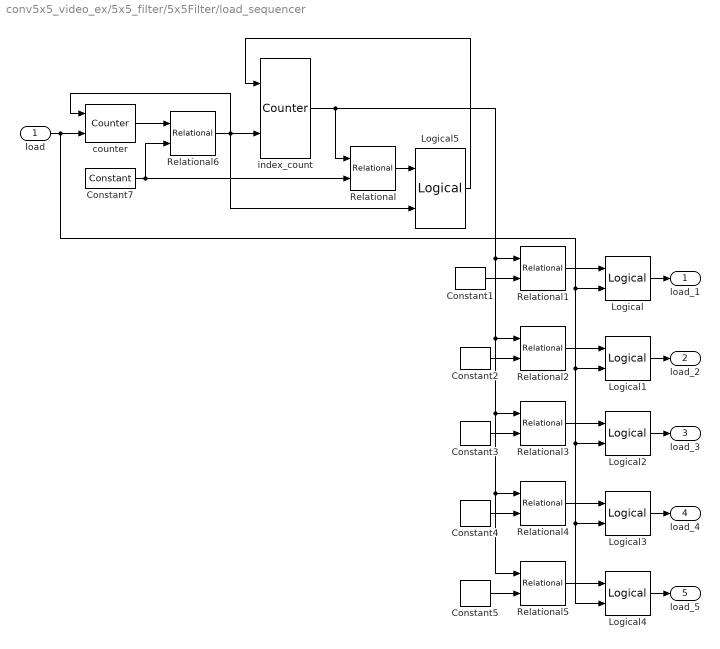
== system conv5x5_video_ex/5x5_filter/5x5Filter/load_sequencer ==
  load : Inport
  Constant1 : xbsIndex_r4/Constant  const=0  gui_display_data_type=Fixed-point  arith_type=Unsigned  n_bits=ceil(log2(num_coef))  bin_pt=0  preci_type=Single  exp_width=8  frac_width=24  explicit_period=off  period=1  equ=P=C  opselect=C  inp2=PCIN>>17  opr=+  inp1=P  carry=CIN  dbl_ovrd=off  block_type=constant
      settings: block_version=VER_STRING_GOES_HERE
  Constant2 : xbsIndex_r4/Constant  const=1  gui_display_data_type=Fixed-point  arith_type=Unsigned  n_bits=ceil(log2(num_coef))  bin_pt=0  preci_type=Single  exp_width=8  frac_width=24  explicit_period=off  period=1  equ=P=C  opselect=C  inp2=PCIN>>17  opr=+  inp1=P  carry=CIN  dbl_ovrd=off  block_type=constant
      settings: block_version=VER_STRING_GOES_HERE
  Constant3 : xbsIndex_r4/Constant  const=2  gui_display_data_type=Fixed-point  arith_type=Unsigned  n_bits=ceil(log2(num_coef))  bin_pt=0  preci_type=Single  exp_width=8  frac_width=24  explicit_period=off  period=1  equ=P=C  opselect=C  inp2=PCIN>>17  opr=+  inp1=P  carry=CIN  dbl_ovrd=off  block_type=constant
      settings: block_version=VER_STRING_GOES_HERE
  Constant4 : xbsIndex_r4/Constant  const=3  gui_display_data_type=Fixed-point  arith_type=Unsigned  n_bits=ceil(log2(num_coef))  bin_pt=0  preci_type=Single  exp_width=8  frac_width=24  explicit_period=off  period=1  equ=P=C  opselect=C  inp2=PCIN>>17  opr=+  inp1=P  carry=CIN  dbl_ovrd=off  block_type=constant
      settings: block_version=VER_STRING_GOES_HERE
  Constant5 : xbsIndex_r4/Constant  const=4  gui_display_data_type=Fixed-point  arith_type=Unsigned  n_bits=ceil(log2(num_coef))  bin_pt=0  preci_type=Single  exp_width=8  frac_width=24  explicit_period=off  period=1  equ=P=C  opselect=C  inp2=PCIN>>17  opr=+  inp1=P  carry=CIN  dbl_ovrd=off  block_type=constant
      settings: block_version=VER_STRING_GOES_HERE
  Constant7 : xbsIndex_r4/Constant  const=num_coef-1  gui_display_data_type=Fixed-point  arith_type=Unsigned  n_bits=ceil(log2(num_coef))  bin_pt=0  preci_type=Single  exp_width=8  frac_width=24  explicit_period=off  period=1  equ=P=C  opselect=C  inp2=PCIN>>17  opr=+  inp1=P  carry=CIN  dbl_ovrd=off  block_type=constant
      settings: block_version=VER_STRING_GOES_HERE
  Logical{,1..5} (6 alike) : xbsIndex_r4/Logical  logical_function=AND  inputs=2  en=off  latency=0  precision=Full  arith_type=Unsigned  n_bits=8  bin_pt=2  align_bp=on  dbl_ovrd=off  block_type=logical
      settings: xl_area=[0, 0, 0, 0, 0, 0, 0]  block_version=VER_STRING_GOES_HERE
  Relational{,1..6} (7 alike) : xbsIndex_r4/Relational  mode=a=b  en=off  latency=0  dbl_ovrd=off  block_type=relational
      settings: xl_area=[0, 0, 0, 0, 0, 0, 0]  block_version=VER_STRING_GOES_HERE
  counter : xbsIndex_r4/Counter  cnt_type=Count Limited  cnt_to=num_coef-1  operation=Up  start_count=0  cnt_by_val=1  arith_type=Unsigned  n_bits=ceil(log2(num_coef))  bin_pt=0  load_pin=off  rst=on  en=on  explicit_period=on  period=1/num_coef  dbl_ovrd=off  use_behavioral_HDL=off  implementation=Fabric  use_rpm=off  block_type=counter
      settings: infoedit="Configurable up, down and up/down counter.<P><P>Hardware notes: Free running counters are the least expensive in hardware.  A count limited counter is implemented by combining a counter with a comparator."  xl_area=[0, 0, 0, 0, 0, 0, 0]  block_version=VER_STRING_GOES_HERE
  index_count : xbsIndex_r4/Counter  cnt_type=Count Limited  cnt_to=num_coef-1  operation=Up  start_count=0  cnt_by_val=1  arith_type=Unsigned  n_bits=ceil(log2(num_coef))  bin_pt=0  load_pin=off  rst=on  en=on  explicit_period=on  period=1/num_coef  dbl_ovrd=off  use_behavioral_HDL=off  implementation=Fabric  use_rpm=off  block_type=counter
      settings: infoedit="Configurable up, down and up/down counter.<P><P>Hardware notes: Free running counters are the least expensive in hardware.  A count limited counter is implemented by combining a counter with a comparator."  xl_area=[0, 0, 0, 0, 0, 0, 0]  block_version=VER_STRING_GOES_HERE
  load_1 : Outport
  load_2 : Outport  Port=2
  load_3 : Outport  Port=3
  load_4 : Outport  Port=4
  load_5 : Outport  Port=5
  wires:
  Constant1/1 -> Relational1/2
  Relational1/1 -> Logical/1
  Logical/1 -> load_1/1
  Constant2/1 -> Relational2/2
  Logical1/1 -> load_2/1
  Relational2/1 -> Logical1/1
  Constant3/1 -> Relational3/2
  Logical2/1 -> load_3/1
  Relational3/1 -> Logical2/1
  Constant4/1 -> Relational4/2
  Logical3/1 -> load_4/1
  Relational4/1 -> Logical3/1
  Constant5/1 -> Relational5/2
  Logical4/1 -> load_5/1
  Relational5/1 -> Logical4/1
  load/1 -> counter/2, Logical/2, Logical1/2, Logical2/2, Logical3/2, Logical4/2
  counter/1 -> Relational6/1
  Constant7/1 -> Relational6/2, Relational/2
  Relational6/1 -> index_count/2, counter/1, Logical5/2
  index_count/1 -> Relational/1, Relational1/1, Relational2/1, Relational3/1, Relational4/1, Relational5/1
  Relational/1 -> Logical5/1
  Logical5/1 -> index_count/1
